simulink library "Hot_Water_EU_TappingCycle"  (R2018b)
settings: Solver=ode45  StartTime=0.0  StopTime=10.0  RelTol=1e-3  EnableMultiTasking=on
undefined symbols (not defined in the file): L
libraries: carnot x4
settings Model: Creator=lena.frank  LastModifiedBy=P41573
settings DataIOCC: LimitDataPoints=on  SaveFormat=Array  SignalLoggingSaveFormat=ModelDataLogs
settings OptimizationCC: ExpressionDepthLimit=2147483647  LifeSpan=inf
settings DebuggingCC: UnderspecifiedInitializationDetection=Classic  MergeDetectMultiDrivingBlocksExec=none  SolverPrmCheckMsg=warning  FcnCallInpInsideContextMsg=warning  StateNameClashWarn=warning  SFUnexpectedBacktrackingDiag=warning  SFNoUnconditionalDefaultTransitionDiag=warning  SFExecutionAtInitializationDiag=none
settings HardwareCC: ProdBitPerPointer=32  ProdBitPerSizeT=32  ProdBitPerPtrDiffT=32  ProdLargestAtomicFloat=None  ProdIntDivRoundTo=Undefined  ProdEndianess=Unspecified  ProdWordSize=32  ProdHWDeviceType=32-bit Generic
settings ModelReferenceCC: PropagateSignalLabelsOutOfModel=off
settings SFSimCC: SimUseLocalCustomCode=off
settings RTWCC: RTWUseLocalCustomCode=off
settings CodeAppCC: StateflowObjectComments=on
settings GRTTargetCC: TargetLangStandard=C89/C90 (ANSI)  GeneratePreprocessorConditionals=Disable all  CombineOutputUpdateFcns=off  GRTInterface=on
settings ConfigComp: CovMetricSettings=dw  CovHtmlReporting=on  CovSaveCumulativeToWorkspaceVar=on  CovSaveSingleToWorkspaceVar=on  CovExternalEMLEnable=off

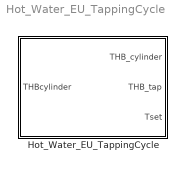
== system Hot_Water_EU_TappingCycle ==
  Hot_Water_EU_TappingCycle : Subsystem  mask(European tapping cycles){T_cold_water=10, eu_tap=L, dTbias=0}
      mask prompts: T_cold_water "Temperature of the cold water"; eu_tap "Tapping cycle"; dTbias "Bias on setpoint temperature in K"
      mask help:
      | Domestic hot water consumption defined by the European Tapping Cycles. This block uses the DHW_Energy_Tapping block.
      | The hot water of the cylinder entering the block is mixed with the cold water to reach the temperature setpoint. The necessary massflow through the cylinder is calculated by this block and set in the outport to the cylinder.
      | The check of mean temperature Tm and peak temperature Tp must be done in a post treatment of the simulation data. A bias on the setpoint temperature can be defined. This assures that the tapping temperature is above the (minimum) setpoint given by the tapping cycle.
      mask Help: web(fullfile(path_carnot('help'),'HotWaterEuTappingCycle.html'),'-helpbrowser')
      mask TypeOptions T_cold_water: T_cold_water/Value
      mask TypeOptions eu_tap: EU_Tapping_Cycle/eu_tap
      mask TypeOptions dTbias: EU_Tapping_Cycle/dTbias
      mask Display:
      | text(15,120,'European Tapping Cycle')
      | plot(0,0,140,130,[70,76,78,63,65,70,70,10],[80,78,74,74,78,80,100,100],[23,23,20,10],[43,47,50,50],[10,10,20,28,30,10],[30,20,20,23,30,30],[22,17],[54,54],[20,20],[54,50],[90,90,50,50],[10,-0,-0,10],[63,64],[60,72],[61,62],[38,50],[60,61],[13,27],[90,85,81,76,70,65,59,54,50],[6,4,6,4,6,4,5,3,5],[68,69],[56,68],[68,68],[32,44],[67,67],[13,23],[73,73],[61,71],[73,73],[43,52],[74,73],[21,36],[78,77],[56,67],[79,79],[34,45],[78,77],[9,23],[82,81],[14,26])

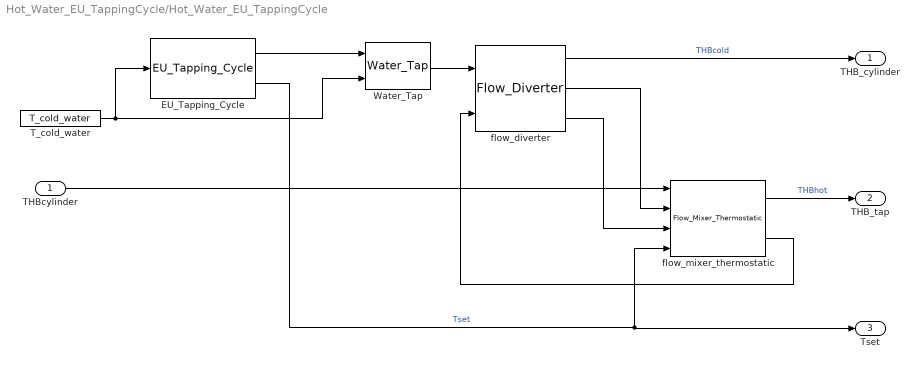
== system Hot_Water_EU_TappingCycle/Hot_Water_EU_TappingCycle ==
  THBcylinder : Inport
  EU_Tapping_Cycle : carnot/Load/Hot_Water_Tapping/EU_Tapping_Cycle  eu_tap=L  dTbias=dTbias
      settings: SourceProductName=Carnot
  T_cold_water : Constant  Value=T_cold_water
  Water_Tap : carnot/Load/Hot_Water_Tapping/Water_Tap  dia=0.02  p=2e5
      settings: SourceProductName=Carnot
  flow_diverter : carnot/Hydraulics/Flow_Diverter
      settings: SourceProductName=Carnot
  flow_mixer_thermostatic : carnot/Hydraulics/Flow_Mixer_Thermostatic  t=1
      settings: SourceProductName=Carnot
  THB_cylinder : Outport
  THB_tap : Outport  Port=2
  Tset : Outport  Port=3
  wires:
  Water_Tap/1 -> flow_diverter/1
  flow_mixer_thermostatic/2 -> flow_diverter/2
  THBcylinder/1 -> flow_mixer_thermostatic/1
  flow_diverter/1 -> THB_cylinder/1  "THBcold"
  flow_diverter/2 -> flow_mixer_thermostatic/2
  flow_diverter/3 -> flow_mixer_thermostatic/3
  T_cold_water/1 -> Water_Tap/2, EU_Tapping_Cycle/1
  EU_Tapping_Cycle/2 -> Tset/1, flow_mixer_thermostatic/4  "Tset"
  EU_Tapping_Cycle/1 -> Water_Tap/1
  flow_mixer_thermostatic/1 -> THB_tap/1  "THBhot"
